simulink subsystem "execute_command_cgn"  (R2025b)
settings: Solver=VariableStepAuto  StartTime=0.0  StopTime=10.0  RelTol=1e-3
undefined symbols (not defined in the file or in its folder): dt_control
settings Model: Creator=vulcangrip  LastModifiedBy=vulcangrip

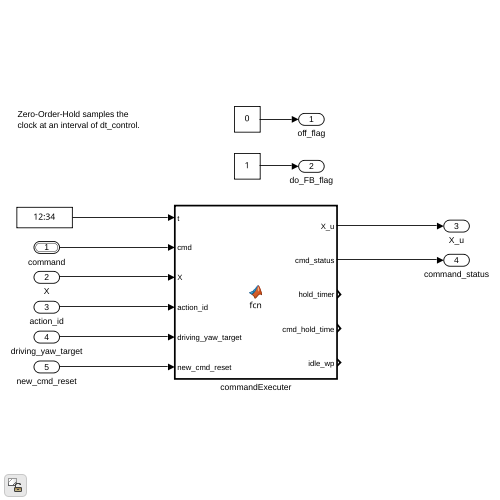
[thumbnail: Simulink's stored preview of the top-level diagram]
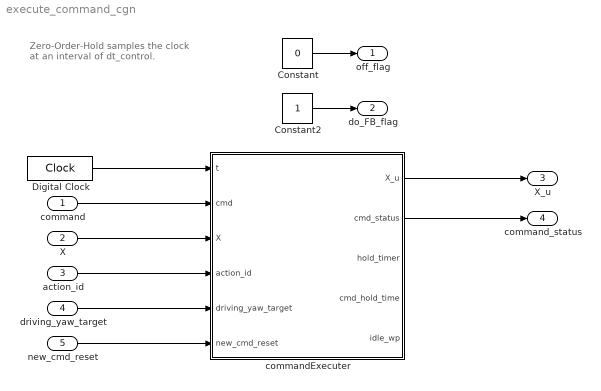
== system execute_command_cgn ==
  note: Zero-Order-Hold samples the
      | clock at an interval of dt_control.
  command : Inport  OutDataTypeStr=Bus: cmd_bus  SampleTime=dt_control
  X : Inport  Port=2  SampleTime=dt_control
  action_id : Inport  Port=3  SampleTime=dt_control
  driving_yaw_target : Inport  Port=4  SampleTime=dt_control
  new_cmd_reset : Inport  Port=5  SampleTime=dt_control
  Constant : Constant  Value=0
  Constant2 : Constant
  Digital Clock : DigitalClock  SampleTime=dt_control
  commandExecuter : MATLAB Function  TreatAsAtomicUnit=on
  off_flag : Outport
  do_FB_flag : Outport  Port=2
  X_u : Outport  Port=3
  command_status : Outport  Port=4
  wires:
  new_cmd_reset/1 -> commandExecuter/6(new_cmd_reset)
  command/1 -> commandExecuter/2(cmd)
  driving_yaw_target/1 -> commandExecuter/5(driving_yaw_target)
  commandExecuter/2(cmd_status) -> command_status/1
  commandExecuter/1(X_u) -> X_u/1
  action_id/1 -> commandExecuter/4(action_id)
  X/1 -> commandExecuter/3(X)
  Constant/1 -> off_flag/1
  Constant2/1 -> do_FB_flag/1
  Digital Clock/1 -> commandExecuter/1(t)

== matlab function execute_command_cgn/commandExecuter ==
  settings: updateMethod=DISCRETE  sampleTime=dt_control
  data: X_u output size=[13 1]; cmd_status output int8 size=[4 1]; hold_timer output; cmd_hold_time output; idle_wp output; t input; cmd input; X input; action_id input; driving_yaw_target input; new_cmd_reset input
function [X_u, cmd_status, hold_timer, cmd_hold_time, idle_wp]  = fcn(t, cmd, X, action_id, driving_yaw_target,new_cmd_reset)

[X_u, cmd_status, hold_timer, cmd_hold_time, idle_wp] = commandExecuter(t, cmd, X, action_id, driving_yaw_target,new_cmd_reset);
